simulink library "EnergyMeter_HC"  (R2018b)
settings: Solver=ode45  StartTime=0.0  StopTime=10.0  RelTol=1e-3  EnableMultiTasking=on
libraries: carnot x1
settings Model: Creator=lena.frank  LastModifiedBy=drhf
settings DataIOCC: LimitDataPoints=on  SaveFormat=Array  SignalLoggingSaveFormat=ModelDataLogs
settings OptimizationCC: ExpressionDepthLimit=2147483647  LifeSpan=inf
settings DebuggingCC: UnderspecifiedInitializationDetection=Classic  MergeDetectMultiDrivingBlocksExec=none  SolverPrmCheckMsg=warning  FcnCallInpInsideContextMsg=warning  StateNameClashWarn=warning  SFUnexpectedBacktrackingDiag=warning  SFNoUnconditionalDefaultTransitionDiag=warning  SFExecutionAtInitializationDiag=none
settings HardwareCC: ProdBitPerPointer=32  ProdBitPerSizeT=32  ProdBitPerPtrDiffT=32  ProdLargestAtomicFloat=None  ProdIntDivRoundTo=Undefined  ProdEndianess=Unspecified  ProdWordSize=32  ProdHWDeviceType=32-bit Generic
settings ModelReferenceCC: PropagateSignalLabelsOutOfModel=off
settings SFSimCC: SimUseLocalCustomCode=off
settings RTWCC: RTWUseLocalCustomCode=off
settings CodeAppCC: StateflowObjectComments=on
settings GRTTargetCC: TargetLangStandard=C89/C90 (ANSI)  GeneratePreprocessorConditionals=Disable all  CombineOutputUpdateFcns=off  GRTInterface=on
settings ConfigComp: CovMetricSettings=dw  CovHtmlReporting=on  CovSaveCumulativeToWorkspaceVar=on  CovSaveSingleToWorkspaceVar=on  CovExternalEMLEnable=off

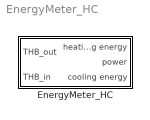
== system EnergyMeter_HC ==
  EnergyMeter_HC : Subsystem  mask(energy meter Heating/Cooling){}
      mask help:
      | Calculates the power and energy of a fluid flow between inlet and outlet of components.
      | Positive power is integrated to the heating energy, negative power is integrated to the cooling energy.
      mask Help: eval('htmlhelp (''chap_4_2e.htm#energy_meter'')');

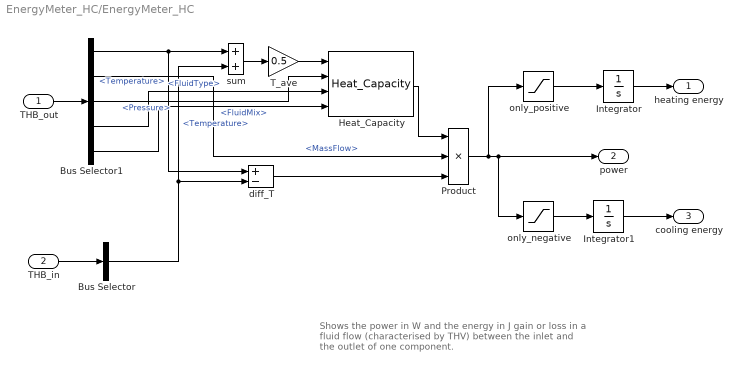
== system EnergyMeter_HC/EnergyMeter_HC ==
  note: Shows the power in W and the energy in J gain or loss
      | in a fluid flow (characterised by THV) between the
      | inlet and the outlet of one component.
  THB_out : Inport
  THB_in : Inport  Port=2
  Bus Selector : BusSelector  OutputSignals=Temperature
  Bus Selector1 : BusSelector  OutputSignals=Temperature,MassFlow,Pressure,FluidType,FluidMix
  Heat_Capacity : carnot/Basic/Material_Properties/Heat_Capacity  VariantControl=CarlibClassic  INPUTARGUMENTS=state variables (classic)  DEBUGLEVEL=DEBUGLEVEL  MAXTOTALWARNINGS=inf  MAXCONSECUTIVEWARNINGS=inf  WRITETOFILE=0  FILENAME='errors.txt'
      settings: SourceProductName=Carnot
  Integrator : Integrator  UpperSaturationLimit=1  LowerSaturationLimit=0
  Integrator1 : Integrator  UpperSaturationLimit=1  LowerSaturationLimit=0
  Product : Product  Inputs=***  SaturateOnIntegerOverflow=on  RndMeth=Zero  InputSameDT=on  OutDataTypeStr=Inherit: Same as first input
  T_ave : Gain  Gain=0.5  SaturateOnIntegerOverflow=on  OutDataTypeStr=Inherit: Same as input  ParamDataTypeStr=Inherit: Same as input
  diff_T : Sum  Inputs=+-  SaturateOnIntegerOverflow=on  InputSameDT=on  OutDataTypeStr=Inherit: Same as first input
  only_negative : Saturate  UpperLimit=0  LowerLimit=-inf
  only_positive : Saturate  UpperLimit=inf  LowerLimit=0
  sum : Sum  SaturateOnIntegerOverflow=on  InputSameDT=on  OutDataTypeStr=Inherit: Same as first input
  heating energy : Outport  InitialOutput=0
  power : Outport  Port=2  InitialOutput=0
  cooling energy : Outport  Port=3  InitialOutput=0
  wires:
  only_positive/1 -> Integrator/1
  only_negative/1 -> Integrator1/1
  Product/1 -> only_positive/1, only_negative/1, power/1
  Integrator1/1 -> cooling energy/1
  Bus Selector1/3 -> Heat_Capacity/2  "<Pressure>"
  T_ave/1 -> Heat_Capacity/1
  sum/1 -> T_ave/1
  Bus Selector/1 -> sum/2, diff_T/2  "<Temperature>"
  diff_T/1 -> Product/3
  Bus Selector1/2 -> Product/2  "<MassFlow>"
  Integrator/1 -> heating energy/1
  Heat_Capacity/1 -> Product/1
  Bus Selector1/5 -> Heat_Capacity/4  "<FluidMix>"
  Bus Selector1/4 -> Heat_Capacity/3  "<FluidType>"
  Bus Selector1/1 -> sum/1, diff_T/1  "<Temperature>"
  THB_out/1 -> Bus Selector1/1
  THB_in/1 -> Bus Selector/1
